simulink subsystem "VehicleElectroThermalLowTemp"  (R2024b)
settings: Solver=VariableStepAuto  StartTime=0.0  StopTime=10.0  RelTol=1e-3
undefined symbols (not defined in the file): battery, coolant_pipe_D, coolant_valve_D_ratio_max, coolant_valve_D_ratio_min, coolant_valve_displacement, vehicleThermal
libraries: fl_lib x64, nesl_utility x23, SimscapeFluids_lib x11, BatteryCurrentManagement x1, ee_lib x1
(part 3 of 3)

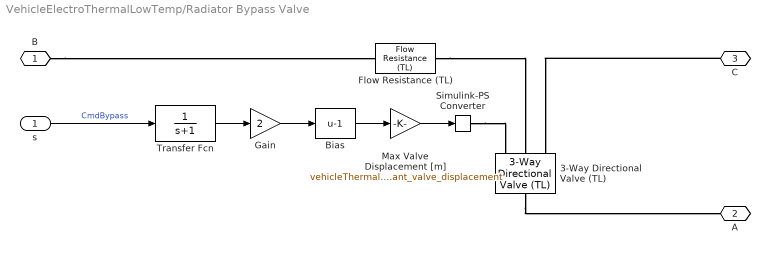
== system VehicleElectroThermalLowTemp/Radiator Bypass Valve ==
  s : Inport
  3-Way Directional Valve (TL) : SimscapeFluids_lib/Thermal Liquid/Valves & Orifices/Directional Control Valves/3-Way Directional Valve (TL)  open_orifices_pos=fluids.thermal_liquid.valves.directional_control_valves.enum.OpenOrifices3Way.PA  open_orifices_neg=fluids.thermal_liquid.valves.directional_control_valves.enum.OpenOrifices3Way.AT  area_spec=fluids.thermal_liquid.valves.directional_control_valves.enum.area_spec.identical  valve_spec=fluids.thermal_liquid.valves.enum.orifice_spec.linear  del_S_max=vehicleThermal.coolant_valve_displacement-(vehicleThermal.coolant_valve_displacement)*(pi * (vehicleThermal.coolant_valve_D_ratio_min*vehicleThermal.coolant_pipe_D)^2 / 4)/(pi * (vehicleThermal.coolant_valve_D_ratio_max*vehicleThermal.coolant_pipe_D)^2 / 4) m  area_max=pi * (vehicleThermal.coolant_valve_D_ratio_max*vehicleThermal.coolant_pipe_D)^2 / 4 m^2  del_S_TLU=[0 0.002 0.004 0.007 0.017] m  valve_area_TLU=[1e-09, 2.0352e-07, 4.0736e-05, .00011438, .00034356] m^2  del_S_flow_TLU=[0 0.002 0.004 0.007 0.017] m  p_diff_TLU=[-.1, .3, .5, .7] MPa  vol_flow_TLU=1e-3 * [1.7e-05, 2e-05, 2.6e-05; .0035, .0045, .0053; .7, .9, 1.06; 1.96, 2.5, 3; 6, 7.7, 9.13] m^3/s  mdot_TLU=[-1e-05, 1.7e-05, 2e-05, 2.6e-05; -.002, .0035, .0045, .0053; -.4, .7, .9, 1.06; -1.13, 1.96, 2.5, 3; -3.45, 6, 7.7, 9.13] kg/s  T_ref_in=293.15 K  p_ref_in=0.101325 MPa  area_leak=pi * (vehicleThermal.coolant_valve_D_ratio_min*vehicleThermal.coolant_pipe_D)^2 / 4 m^2  Cd=0.7  Re_c=12  smoothing_factor=0.01  pressure_recovery=simscape.enum.onoff.on  area=pi * vehicleThermal.coolant_pipe_D^2 / 4 m^2  S_max_PA=(vehicleThermal.coolant_valve_displacement)*(pi * (vehicleThermal.coolant_valve_D_ratio_min*vehicleThermal.coolant_pipe_D)^2 / 4)/(pi * (vehicleThermal.coolant_valve_D_ratio_max*vehicleThermal.coolant_pipe_D)^2 / 4) - (vehicleThermal.coolant_valve_offset) + vehicleThermal.coolant_valve_displacement-(vehicleThermal.coolant_valve_displacement)*(pi * (vehicleThermal.coolant_valve_D_ratio_min*vehicleThermal.coolant_pipe_D)^2 / 4)/(pi * (vehicleThermal.coolant_valve_D_ratio_max*vehicleThermal.coolant_pipe_D)^2 / 4) m  del_S_max_PA=coolant_valve_displacement-(coolant_valve_displacement)*(pi * (coolant_valve_D_ratio_min*coolant_pipe_D)^2 / 4)/(pi * (coolant_valve_D_ratio_max*coolant_pipe_D)^2 / 4) m  area_max_PA=pi * (coolant_valve_D_ratio_max*coolant_pipe_D)^2 / 4 m^2  del_S_TLU_PA=[0 0.002 0.004 0.007 0.017] m  valve_area_TLU_PA=[1e-09, 2.0352e-07, 4.0736e-05, .00011438, .00034356] m^2  del_S_flow_TLU_PA=[0 0.002 0.004 0.007 0.017] m  p_diff_TLU_PA=[-.1, .3, .5, .7] MPa  vol_flow_TLU_PA=1e-3 * [1.7e-05, 2e-05, 2.6e-05; .0035, .0045, .0053; .7, .9, 1.06; 1.96, 2.5, 3; 6, 7.7, 9.13] m^3/s  mdot_TLU_PA=[-1e-05, 1.7e-05, 2e-05, 2.6e-05; -.002, .0035, .0045, .0053; -.4, .7, .9, 1.06; -1.13, 1.96, 2.5, 3; -3.45, 6, 7.7, 9.13] kg/s  S_max_AT=-(vehicleThermal.coolant_valve_displacement)*(pi * (vehicleThermal.coolant_valve_D_ratio_min*vehicleThermal.coolant_pipe_D)^2 / 4)/(pi * (vehicleThermal.coolant_valve_D_ratio_max*vehicleThermal.coolant_pipe_D)^2 / 4) + (vehicleThermal.coolant_valve_offset) - (vehicleThermal.coolant_valve_displacement-(vehicleThermal.coolant_valve_displacement)*(pi * (vehicleThermal.coolant_valve_D_ratio_min*vehicleThermal.coolant_pipe_D)^2 / 4)/(pi * (vehicleThermal.coolant_valve_D_ratio_max*vehicleThermal.coolant_pipe_D)^2 / 4)) m  del_S_max_AT=coolant_valve_displacement-(coolant_valve_displacement)*(pi * (coolant_valve_D_ratio_min*coolant_pipe_D)^2 / 4)/(pi * (coolant_valve_D_ratio_max*coolant_pipe_D)^2 / 4) m  area_max_AT=pi * (coolant_valve_D_ratio_max*coolant_pipe_D)^2 / 4 m^2  del_S_TLU_AT=[0 0.002 0.004 0.007 0.017] m  valve_area_TLU_AT=[1e-09, 2.0352e-07, 4.0736e-05, .00011438, .00034356] m^2  del_S_flow_TLU_AT=[0 0.002 0.004 0.007 0.017] m  p_diff_TLU_AT=[-.1, .3, .5, .7] MPa  vol_flow_TLU_AT=1e-3 * [1.7e-05, 2e-05, 2.6e-05; .0035, .0045, .0053; .7, .9, 1.06; 1.96, 2.5, 3; 6, 7.7, 9.13] m^3/s  mdot_TLU_AT=[-1e-05, 1.7e-05, 2e-05, 2.6e-05; -.002, .0035, .0045, .0053; -.4, .7, .9, 1.06; -1.13, 1.96, 2.5, 3; -3.45, 6, 7.7, 9.13] kg/s  S_max_PT=2.5e-3 m  del_S_max_PT=0.005 m  area_max_PT=1e-4 m^2  del_S_TLU_PT=[0, .002, .004, .007, .017] m  valve_area_TLU_PT=[1e-09, 2.0352e-07, 4.0736e-05, .00011438, .00034356] m^2  del_S_flow_TLU_PT=[0, .002, .004, .007, .017] m  p_diff_TLU_PT=[.3, .5, .7] MPa  vol_flow_TLU_PT=1e-3 * [1.7e-05, 2e-05, 2.6e-05; .0035, .0045, .0053; .7, .9, 1.06; 1.96, 2.5, 3; 6, 7.7, 9.13] m^3/s  mdot_TLU_PT=[1.7e-05, 2e-05, 2.6e-05; .0035, .0045, .0053; .7, .9, 1.06; 1.96, 2.5, 3; 6, 7.7, 9.13] kg/s
      settings: InternalSimscapePortConfiguration="{\"Bottom\":[],\"Left\":[{\"id\":\"A\",\"label\":\"A\",\"type\":\"foundation.thermal_liquid.thermal_liquid\"}],\"Right\":[{\"id\":\"S\",\"label\":\"S\",\"type\":\"input\"},{\"id\":\"P\",\"label\":\"P\",\"type\":\"foundation.thermal_liquid.thermal_liquid\"},{\"id\":\"T\",\"label\":\"T\",\"type\":\"foundation.thermal_liquid.thermal_liquid\"}],\"Top\":[]}"
  Bias : Bias  Bias=-1  SaturateOnIntegerOverflow=off
  Flow Resistance (TL) : fl_lib/Thermal Liquid/Elements/Flow Resistance (TL)  delta_p_nominal=0.001 MPa  mdot_nominal=0.3 kg/s  area=pi * vehicleThermal.coolant_pipe_D^2 / 4 m^2  laminar_fraction=1e-3
  Gain : Gain  Gain=2
  Max Valve Displacement [m] : Gain  Gain=vehicleThermal.coolant_valve_displacement
  Simulink-PS Converter : nesl_utility/Simulink-PS Converter  PhysicalDomain=network_engine_domain  SubClassName=ps_input  LeftPortType=input  RightPortType=output  PseudoPeriodic=off  Frequencies=[]  NoiseDistribution=none  NoiseParameters=[]  Unit=m  AffineConversion=off  FilteringAndDerivatives=provide  SimscapeFilterOrder=1  InputFilterTimeConstant=0.001  UdotUserProvided=0
  Transfer Fcn : TransferFcn  Denominator=[1 1]
  B : PMIOPort  Side=Left
  A : PMIOPort  Port=2  Side=Left
  C : PMIOPort  Port=3  Side=Right
  wires:
  Transfer Fcn/1 -> Gain/1
  Bias/1 -> Max Valve Displacement [m]/1
  s/1 -> Transfer Fcn/1  "CmdBypass"
  Max Valve Displacement [m]/1 -> Simulink-PS Converter/1
  Gain/1 -> Bias/1
  connections:
  Flow Resistance (TL)/LConn1 -- 3-Way Directional Valve (TL)/RConn2
  Simulink-PS Converter/RConn1 -- 3-Way Directional Valve (TL)/RConn1
  C/RConn1 -- 3-Way Directional Valve (TL)/RConn3
  B/RConn1 -- Flow Resistance (TL)/RConn1
  3-Way Directional Valve (TL)/LConn1 -- A/RConn1

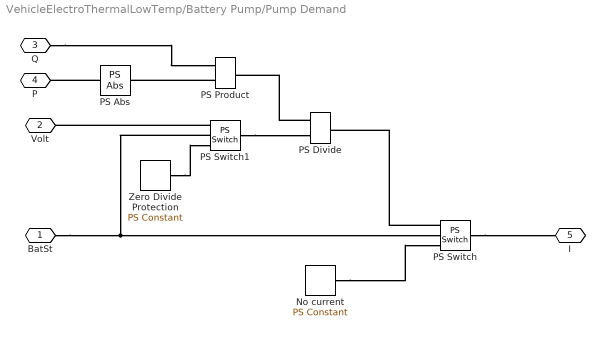
== system VehicleElectroThermalLowTemp/Battery Pump/Pump Demand ==
  No current : fl_lib/Physical Signals/Sources/PS Constant  constant=0 A
  PS Abs : fl_lib/Physical Signals/Nonlinear Operators/PS Abs
      settings: InternalSimscapePortConfiguration="{\"Bottom\":[],\"Left\":[{\"id\":\"I\",\"label\":\"\",\"type\":\"input\"}],\"Right\":[{\"id\":\"O\",\"label\":\"\",\"type\":\"output\"}],\"Top\":[]}"
  PS Divide : fl_lib/Physical Signals/Functions/PS Divide
  PS Product : fl_lib/Physical Signals/Functions/PS Product
  PS Switch : fl_lib/Physical Signals/Nonlinear Operators/PS Switch  Threshold=0.5
      settings: InternalSimscapePortConfiguration="{\"Bottom\":[],\"Left\":[{\"id\":\"I1\",\"label\":\"\",\"type\":\"input\"},{\"id\":\"I2\",\"label\":\"\",\"type\":\"input\"},{\"id\":\"I3\",\"label\":\"\",\"type\":\"input\"}],\"Right\":[{\"id\":\"O\",\"label\":\"\",\"type\":\"output\"}],\"Top\":[]}"
  PS Switch1 : fl_lib/Physical Signals/Nonlinear Operators/PS Switch  Threshold=0.5
      settings: InternalSimscapePortConfiguration="{\"Bottom\":[],\"Left\":[{\"id\":\"I1\",\"label\":\"\",\"type\":\"input\"},{\"id\":\"I2\",\"label\":\"\",\"type\":\"input\"},{\"id\":\"I3\",\"label\":\"\",\"type\":\"input\"}],\"Right\":[{\"id\":\"O\",\"label\":\"\",\"type\":\"output\"}],\"Top\":[]}"
  Zero Divide Protection : fl_lib/Physical Signals/Sources/PS Constant  constant=1 V
  BatSt : PMIOPort  Side=Left
  Volt : PMIOPort  Port=2  Side=Left
  Q : PMIOPort  Port=3  Side=Left
  P : PMIOPort  Port=4  Side=Left
  I : PMIOPort  Port=5  Side=Right
  connections:
  PS Product/LConn2 -- PS Abs/RConn1
  Zero Divide Protection/RConn1 -- PS Switch1/LConn3
  PS Switch1/RConn1 -- PS Divide/LConn2
  PS Abs/LConn1 -- P/RConn1
  Q/RConn1 -- PS Product/LConn1
  PS Divide/LConn1 -- PS Product/RConn1
  PS Switch/RConn1 -- I/RConn1
  PS Switch1/LConn2 -- PS Switch/LConn2 -- BatSt/RConn1
  PS Switch/LConn1 -- PS Divide/RConn1
  PS Switch1/LConn1 -- Volt/RConn1
  No current/RConn1 -- PS Switch/LConn3

== system VehicleElectroThermalLowTemp/Battery Pump/current sensing1 ==
  Current Sensor : fl_lib/Electrical/Electrical Sensors/Current Sensor
  PS-Simulink Converter : nesl_utility/PS-Simulink Converter  PhysicalDomain=network_engine_domain  SubClassName=ps_output  LeftPortType=input  RightPortType=output  PseudoPeriodic=off  Frequencies=[]  VectorFormat=inherit  Unit=inherit  AffineConversion=off
  "  " : PMIOPort  Side=Left
  " " : PMIOPort  Port=2  Side=Right
  "   " : Outport
  wires:
  PS-Simulink Converter/1 -> "   "/1
  connections:
  Current Sensor/RConn2 -- " "/RConn1
  Current Sensor/LConn1 -- "  "/RConn1
  PS-Simulink Converter/LConn1 -- Current Sensor/RConn1

== system VehicleElectroThermalLowTemp/Chiller Bypass Valve/Valve Control ==
  ThCtrl : Inport
  Bias : Bias  Bias=-1  SaturateOnIntegerOverflow=off
  Gain : Gain  Gain=2
  Max Valve Displacement [m] : Gain  Gain=vehicleThermal.coolant_valve_displacement
  Simulink-PS Converter : nesl_utility/Simulink-PS Converter  PhysicalDomain=network_engine_domain  SubClassName=ps_input  LeftPortType=input  RightPortType=output  PseudoPeriodic=off  Frequencies=[]  NoiseDistribution=none  NoiseParameters=[]  Unit=m  AffineConversion=off  FilteringAndDerivatives=provide  SimscapeFilterOrder=1  InputFilterTimeConstant=0.001  UdotUserProvided=0
  Transfer Fcn : TransferFcn  Denominator=[1 1]
  Disp : PMIOPort  Side=Right
  wires:
  Transfer Fcn/1 -> Gain/1
  ThCtrl/1 -> Transfer Fcn/1
  Max Valve Displacement [m]/1 -> Simulink-PS Converter/1
  Bias/1 -> Max Valve Displacement [m]/1
  Gain/1 -> Bias/1
  connections:
  Simulink-PS Converter/RConn1 -- Disp/RConn1

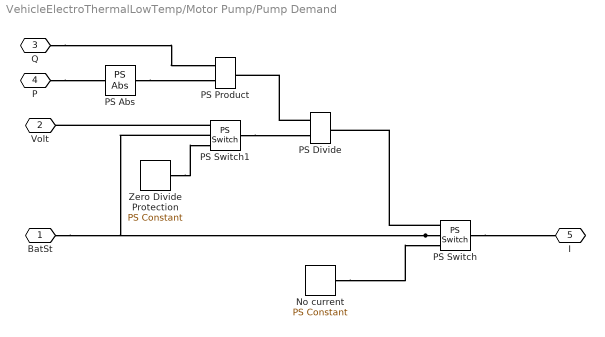
== system VehicleElectroThermalLowTemp/Motor Pump/Pump Demand ==
  No current : fl_lib/Physical Signals/Sources/PS Constant  constant=0 A
  PS Abs : fl_lib/Physical Signals/Nonlinear Operators/PS Abs
      settings: InternalSimscapePortConfiguration="{\"Bottom\":[],\"Left\":[{\"id\":\"I\",\"label\":\"\",\"type\":\"input\"}],\"Right\":[{\"id\":\"O\",\"label\":\"\",\"type\":\"output\"}],\"Top\":[]}"
  PS Divide : fl_lib/Physical Signals/Functions/PS Divide
  PS Product : fl_lib/Physical Signals/Functions/PS Product
  PS Switch : fl_lib/Physical Signals/Nonlinear Operators/PS Switch  Threshold=0.5
      settings: InternalSimscapePortConfiguration="{\"Bottom\":[],\"Left\":[{\"id\":\"I1\",\"label\":\"\",\"type\":\"input\"},{\"id\":\"I2\",\"label\":\"\",\"type\":\"input\"},{\"id\":\"I3\",\"label\":\"\",\"type\":\"input\"}],\"Right\":[{\"id\":\"O\",\"label\":\"\",\"type\":\"output\"}],\"Top\":[]}"
  PS Switch1 : fl_lib/Physical Signals/Nonlinear Operators/PS Switch  Threshold=0.5
      settings: InternalSimscapePortConfiguration="{\"Bottom\":[],\"Left\":[{\"id\":\"I1\",\"label\":\"\",\"type\":\"input\"},{\"id\":\"I2\",\"label\":\"\",\"type\":\"input\"},{\"id\":\"I3\",\"label\":\"\",\"type\":\"input\"}],\"Right\":[{\"id\":\"O\",\"label\":\"\",\"type\":\"output\"}],\"Top\":[]}"
  Zero Divide Protection : fl_lib/Physical Signals/Sources/PS Constant  constant=1 V
  BatSt : PMIOPort  Side=Left
  Volt : PMIOPort  Port=2  Side=Left
  Q : PMIOPort  Port=3  Side=Left
  P : PMIOPort  Port=4  Side=Left
  I : PMIOPort  Port=5  Side=Right
  connections:
  PS Abs/RConn1 -- PS Product/LConn2
  Zero Divide Protection/RConn1 -- PS Switch1/LConn3
  PS Switch1/RConn1 -- PS Divide/LConn2
  Q/RConn1 -- PS Product/LConn1
  P/RConn1 -- PS Abs/LConn1
  PS Divide/LConn1 -- PS Product/RConn1
  PS Switch/RConn1 -- I/RConn1
  PS Switch/LConn2 -- PS Switch1/LConn2 -- BatSt/RConn1
  PS Switch/LConn1 -- PS Divide/RConn1
  PS Switch1/LConn1 -- Volt/RConn1
  No current/RConn1 -- PS Switch/LConn3

== system VehicleElectroThermalLowTemp/Motor Pump/current sensing1 ==
  Current Sensor : fl_lib/Electrical/Electrical Sensors/Current Sensor
  PS-Simulink Converter : nesl_utility/PS-Simulink Converter  PhysicalDomain=network_engine_domain  SubClassName=ps_output  LeftPortType=input  RightPortType=output  PseudoPeriodic=off  Frequencies=[]  VectorFormat=inherit  Unit=inherit  AffineConversion=off
  "  " : PMIOPort  Side=Left
  " " : PMIOPort  Port=2  Side=Right
  "   " : Outport
  wires:
  PS-Simulink Converter/1 -> "   "/1
  connections:
  Current Sensor/RConn2 -- " "/RConn1
  Current Sensor/LConn1 -- "  "/RConn1
  PS-Simulink Converter/LConn1 -- Current Sensor/RConn1

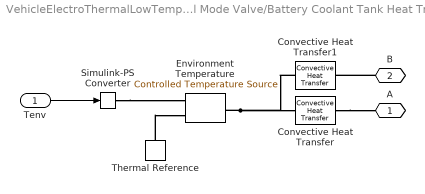
== system VehicleElectroThermalLowTemp/Parallel-Serial Mode Valve/Battery Coolant Tank Heat Transfer ==
  Tenv : Inport
  Convective Heat Transfer : fl_lib/Thermal/Thermal Elements/Convective Heat Transfer  thermal_type=foundation.enum.constant_variable.constant  area=3 * vehicleThermal.coolant_tank_area m^2  heat_tr_coeff=20 W/(m^2 * K)  min_heat_tr_coeff=1e-3 W/(K*m^2)  T_specify=off  T_priority=None  T=0 K  T_nominal_specify=off  T_nominal_value=1  T_nominal_unit=K  Q_specify=off  Q_priority=None  Q=0 W  Q_nominal_specify=off  Q_nominal_value=1  Q_nominal_unit=W
  Convective Heat Transfer1 : fl_lib/Thermal/Thermal Elements/Convective Heat Transfer  thermal_type=foundation.enum.constant_variable.constant  area=3 * vehicleThermal.coolant_tank_area m^2  heat_tr_coeff=20 W/(m^2 * K)  min_heat_tr_coeff=1e-3 W/(K*m^2)  T_specify=off  T_priority=None  T=0 K  T_nominal_specify=off  T_nominal_value=1  T_nominal_unit=K  Q_specify=off  Q_priority=None  Q=0 W  Q_nominal_specify=off  Q_nominal_value=1  Q_nominal_unit=W
  Environment Temperature : fl_lib/Thermal/Thermal Sources/Controlled Temperature Source
  Simulink-PS Converter : nesl_utility/Simulink-PS Converter  PhysicalDomain=network_engine_domain  SubClassName=ps_input  LeftPortType=input  RightPortType=output  PseudoPeriodic=off  Frequencies=[]  NoiseDistribution=none  NoiseParameters=[]  Unit=K  AffineConversion=on  FilteringAndDerivatives=provide  SimscapeFilterOrder=1  InputFilterTimeConstant=0.001  UdotUserProvided=0
  Thermal Reference : fl_lib/Thermal/Thermal Elements/Thermal Reference
  A : PMIOPort  Side=Left
  B : PMIOPort  Port=2  Side=Left
  wires:
  Tenv/1 -> Simulink-PS Converter/1
  connections:
  Convective Heat Transfer/LConn1 -- A/RConn1
  B/RConn1 -- Convective Heat Transfer1/LConn1
  Simulink-PS Converter/RConn1 -- Environment Temperature/RConn1
  Thermal Reference/LConn1 -- Environment Temperature/RConn2
  Environment Temperature/LConn1 -- Convective Heat Transfer1/RConn1 -- Convective Heat Transfer/RConn1

== system VehicleElectroThermalLowTemp/Parallel-Serial Mode Valve/Motor Coolant Tank Heat Transfer ==
  Tenv : Inport
  Convective Heat Transfer : fl_lib/Thermal/Thermal Elements/Convective Heat Transfer  thermal_type=foundation.enum.constant_variable.constant  area=3 * vehicleThermal.coolant_tank_area m^2  heat_tr_coeff=20 W/(m^2 * K)  min_heat_tr_coeff=1e-3 W/(K*m^2)  T_specify=off  T_priority=None  T=0 K  T_nominal_specify=off  T_nominal_value=1  T_nominal_unit=K  Q_specify=off  Q_priority=None  Q=0 W  Q_nominal_specify=off  Q_nominal_value=1  Q_nominal_unit=W
  Convective Heat Transfer1 : fl_lib/Thermal/Thermal Elements/Convective Heat Transfer  thermal_type=foundation.enum.constant_variable.constant  area=3 * vehicleThermal.coolant_tank_area m^2  heat_tr_coeff=20 W/(m^2 * K)  min_heat_tr_coeff=1e-3 W/(K*m^2)  T_specify=off  T_priority=None  T=0 K  T_nominal_specify=off  T_nominal_value=1  T_nominal_unit=K  Q_specify=off  Q_priority=None  Q=0 W  Q_nominal_specify=off  Q_nominal_value=1  Q_nominal_unit=W
  Environment Temperature : fl_lib/Thermal/Thermal Sources/Controlled Temperature Source
  Simulink-PS Converter : nesl_utility/Simulink-PS Converter  PhysicalDomain=network_engine_domain  SubClassName=ps_input  LeftPortType=input  RightPortType=output  PseudoPeriodic=off  Frequencies=[]  NoiseDistribution=none  NoiseParameters=[]  Unit=K  AffineConversion=on  FilteringAndDerivatives=provide  SimscapeFilterOrder=1  InputFilterTimeConstant=0.001  UdotUserProvided=0
  Thermal Reference : fl_lib/Thermal/Thermal Elements/Thermal Reference
  A : PMIOPort  Side=Right
  B : PMIOPort  Port=2  Side=Right
  wires:
  Tenv/1 -> Simulink-PS Converter/1
  connections:
  A/RConn1 -- Convective Heat Transfer/LConn1
  B/RConn1 -- Convective Heat Transfer1/LConn1
  Convective Heat Transfer1/RConn1 -- Environment Temperature/LConn1 -- Convective Heat Transfer/RConn1
  Thermal Reference/LConn1 -- Environment Temperature/RConn2
  Simulink-PS Converter/RConn1 -- Environment Temperature/RConn1

== system VehicleElectroThermalLowTemp/Parallel-Serial Mode Valve/Valve Control ==
  Ctrl : Inport
  Bias : Bias  Bias=-1  SaturateOnIntegerOverflow=off
  Gain : Gain  Gain=2
  Max Valve Displacement [m] : Gain  Gain=vehicleThermal.coolant_valve_displacement
  Simulink-PS Converter : nesl_utility/Simulink-PS Converter  PhysicalDomain=network_engine_domain  SubClassName=ps_input  LeftPortType=input  RightPortType=output  PseudoPeriodic=off  Frequencies=[]  NoiseDistribution=none  NoiseParameters=[]  Unit=m  AffineConversion=off  FilteringAndDerivatives=provide  SimscapeFilterOrder=1  InputFilterTimeConstant=0.001  UdotUserProvided=0
  Transfer Fcn : TransferFcn  Denominator=[1 1]
  disp : PMIOPort  Side=Right
  wires:
  Ctrl/1 -> Transfer Fcn/1
  Max Valve Displacement [m]/1 -> Simulink-PS Converter/1
  Transfer Fcn/1 -> Gain/1
  Gain/1 -> Bias/1
  Bias/1 -> Max Valve Displacement [m]/1
  connections:
  Simulink-PS Converter/RConn1 -- disp/RConn1

== system VehicleElectroThermalLowTemp/Radiator/Fan_Control ==
  VehSpd : Inport
  FanCtrl : Inport  Port=2
  Air Speed Table [m/s] : Lookup_n-D  BreakpointsForDimension1=[0 40 90 110 150 180 198]  BreakpointsForDimension2=[0 14.4]  IndexSearchMethod=Linear search  BeginIndexSearchUsingPreviousIndexResult=on  Table=[0 0.8 2.2 2.7 3.6 4.1 4.6; 1.5 2.3 3.2 3.5 4.3 4.8 5.1]'  InternalRulePriority=Speed  RndMeth=Simplest
      settings: InputPortMap=u0,u1
  Fan Area [m^2] : Gain  Gain=vehicleThermal.fan_area
  Max Fan : Gain  Gain=14.4
  Simulink-PS Converter4 : nesl_utility/Simulink-PS Converter  PhysicalDomain=network_engine_domain  SubClassName=ps_input  LeftPortType=input  RightPortType=output  PseudoPeriodic=off  Frequencies=[]  NoiseDistribution=none  NoiseParameters=[]  Unit=m^3/s  AffineConversion=off  FilteringAndDerivatives=provide  SimscapeFilterOrder=1  InputFilterTimeConstant=0.001  UdotUserProvided=0
  Transfer Fcn : TransferFcn  Denominator=[5 1]
  disp : PMIOPort  Side=Right
  wires:
  Max Fan/1 -> Air Speed Table [m/s]/2
  Transfer Fcn/1 -> Fan Area [m^2]/1
  Air Speed Table [m/s]/1 -> Transfer Fcn/1
  FanCtrl/1 -> Max Fan/1
  VehSpd/1 -> Air Speed Table [m/s]/1
  Fan Area [m^2]/1 -> Simulink-PS Converter4/1
  connections:
  disp/RConn1 -- Simulink-PS Converter4/RConn1

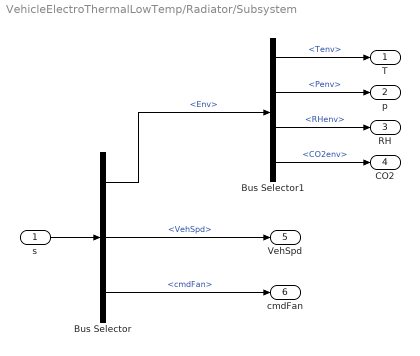
== system VehicleElectroThermalLowTemp/Radiator/Subsystem ==
  s : Inport
  Bus Selector : BusSelector  OutputSignals=Env,VehSpd,cmdFan
  Bus Selector1 : BusSelector  OutputSignals=Tenv,Penv,RHenv,CO2env
  T : Outport
  p : Outport  Port=2
  RH : Outport  Port=3
  CO2 : Outport  Port=4
  VehSpd : Outport  Port=5
  cmdFan : Outport  Port=6
  wires:
  Bus Selector1/4 -> CO2/1  "<CO2env>"
  Bus Selector/2 -> VehSpd/1  "<VehSpd>"
  Bus Selector1/1 -> T/1  "<Tenv>"
  s/1 -> Bus Selector/1
  Bus Selector1/2 -> p/1  "<Penv>"
  Bus Selector/1 -> Bus Selector1/1  "<Env>"
  Bus Selector/3 -> cmdFan/1  "<cmdFan>"
  Bus Selector1/3 -> RH/1  "<RHenv>"
